simulink model "IOControls"  (R2019b)
settings: configuration reference "ConfigSet_IOControls_Reference" (kept outside this file)
model workspace (MAT data in the model file):
  SampleTime = 0.05
libraries: IOStateMachinesLib x274, SignalGeneratorsLib x1, simulink x1
(part 2 of 10)

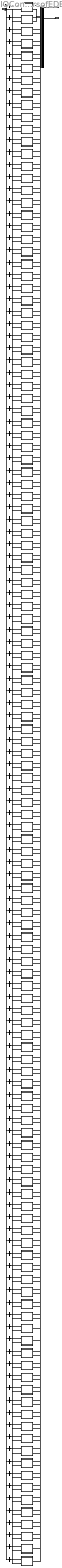
== system IOControls/ForEachVehicle/IOControls/Non-CabControl/CircuitBreakersofEDB ==
  ModelInputs : Inport
  Initialise : Inport  Port=2
  AC1CB : Subsystem  mask{InitState=1, ControlStates=[0,1], OnStateValue=1, OffStateValue=0}
      mask prompts: InitState "Initial State"; ControlStates "Software State Values"; OnStateValue "On State Value"; OffStateValue "Off State Value"
  AC2CB : Subsystem  mask{InitState=1, ControlStates=[0,1], OnStateValue=1, OffStateValue=0}
      mask prompts: InitState "Initial State"; ControlStates "Software State Values"; OnStateValue "On State Value"; OffStateValue "Off State Value"
  ADDCOS : Subsystem  mask{InitState=0, ControlStates=[0,1], OnStateValue=1, OffStateValue=0}
      mask prompts: InitState "Initial State"; ControlStates "Software State Values"; OnStateValue "On State Value"; OffStateValue "Off State Value"
  APSCB : Subsystem  mask{InitState=1, ControlStates=[0,1], OnStateValue=1, OffStateValue=0}
      mask prompts: InitState "Initial State"; ControlStates "Software State Values"; OnStateValue "On State Value"; OffStateValue "Off State Value"
  APSICB : Subsystem  mask{InitState=1, ControlStates=[0,1], OnStateValue=1, OffStateValue=0}
      mask prompts: InitState "Initial State"; ControlStates "Software State Values"; OnStateValue "On State Value"; OffStateValue "Off State Value"
  BCBCB : Subsystem  mask{InitState=1, ControlStates=[0,1], OnStateValue=1, OffStateValue=0}
      mask prompts: InitState "Initial State"; ControlStates "Software State Values"; OnStateValue "On State Value"; OffStateValue "Off State Value"
  BCGCB : Subsystem  mask{InitState=1, ControlStates=[0,1], OnStateValue=1, OffStateValue=0}
      mask prompts: InitState "Initial State"; ControlStates "Software State Values"; OnStateValue "On State Value"; OffStateValue "Off State Value"
  BC_Inputs : BusCreator  Inputs=128
  BC_MCBTrip : BusCreator  Inputs=124
  BECUCB1 : Subsystem  mask{InitState=1, ControlStates=[0,1], OnStateValue=1, OffStateValue=0}
      mask prompts: InitState "Initial State"; ControlStates "Software State Values"; OnStateValue "On State Value"; OffStateValue "Off State Value"
  BECUCB2 : Subsystem  mask{InitState=1, ControlStates=[0,1], OnStateValue=1, OffStateValue=0}
      mask prompts: InitState "Initial State"; ControlStates "Software State Values"; OnStateValue "On State Value"; OffStateValue "Off State Value"
  BECUCB3 : Subsystem  mask{InitState=1, ControlStates=[0,1], OnStateValue=1, OffStateValue=0}
      mask prompts: InitState "Initial State"; ControlStates "Software State Values"; OnStateValue "On State Value"; OffStateValue "Off State Value"
  BLCB : Subsystem  mask{InitState=1, ControlStates=[0,1], OnStateValue=1, OffStateValue=0}
      mask prompts: InitState "Initial State"; ControlStates "Software State Values"; OnStateValue "On State Value"; OffStateValue "Off State Value"
  BS_Control1 : BusSelector  OutputSignals=EBLR2CB
  BS_Control10 : BusSelector  OutputSignals=ILCB1
  BS_Control100 : BusSelector  OutputSignals=SP3CB
  BS_Control101 : BusSelector  OutputSignals=SP4CB
  BS_Control102 : BusSelector  OutputSignals=SP5CB
  BS_Control103 : BusSelector  OutputSignals=SPCB6
  BS_Control104 : BusSelector  OutputSignals=SPCB7
  BS_Control105 : BusSelector  OutputSignals=SPCB8
  BS_Control106 : BusSelector  OutputSignals=RPTCB
  BS_Control107 : BusSelector  OutputSignals=TERCB1
  BS_Control108 : BusSelector  OutputSignals=TERCB2
  BS_Control109 : BusSelector  OutputSignals=SPSW
  BS_Control11 : BusSelector  OutputSignals=ILCB2
  BS_Control110 : BusSelector  OutputSignals=SPPB
  BS_Control111 : BusSelector  OutputSignals=APSCB
  BS_Control112 : BusSelector  OutputSignals=APSICB
  BS_Control113 : BusSelector  OutputSignals=BCGCB
  BS_Control114 : BusSelector  OutputSignals=DSCB
  BS_Control115 : BusSelector  OutputSignals=MTBMCCB
  BS_Control116 : BusSelector  OutputSignals=PADCB
  BS_Control117 : BusSelector  OutputSignals=PANCB
  BS_Control118 : BusSelector  OutputSignals=SSCB
  BS_Control119 : BusSelector  OutputSignals=PTCB
  BS_Control12 : BusSelector  OutputSignals=LDICB
  BS_Control120 : BusSelector  OutputSignals=VCBCB
  BS_Control121 : BusSelector  OutputSignals=SP12CB
  BS_Control122 : BusSelector  OutputSignals=MTBM1CB
  BS_Control123 : BusSelector  OutputSignals=MTBM2CB
  BS_Control124 : BusSelector  OutputSignals=SP11CB
  BS_Control125 : BusSelector  OutputSignals=SP6CB
  BS_Control126 : BusSelector  OutputSignals=MTOPCB
  BS_Control127 : BusSelector  OutputSignals=ORDCOS
  BS_Control128 : BusSelector  OutputSignals=ADDCOS
  BS_Control13 : BusSelector  OutputSignals=LDLCB
  BS_Control14 : BusSelector  OutputSignals=LDRCB
  BS_Control15 : BusSelector  OutputSignals=MLCB
  BS_Control16 : BusSelector  OutputSignals=MMCB
  BS_Control17 : BusSelector  OutputSignals=NBCB
  BS_Control18 : BusSelector  OutputSignals=NVICB
  BS_Control19 : BusSelector  OutputSignals=OCCB1
  BS_Control2 : BusSelector  OutputSignals=EBMVCB
  BS_Control20 : BusSelector  OutputSignals=OCCB2
  BS_Control21 : BusSelector  OutputSignals=ODDCB
  BS_Control22 : BusSelector  OutputSignals=PBCB
  BS_Control23 : BusSelector  OutputSignals=PISCB1
  BS_Control24 : BusSelector  OutputSignals=PISCB2
  BS_Control25 : BusSelector  OutputSignals=POCB
  BS_Control26 : BusSelector  OutputSignals=PPU1CB
  BS_Control27 : BusSelector  OutputSignals=PPU2CB
  BS_Control28 : BusSelector  OutputSignals=PPU3CB
  BS_Control29 : BusSelector  OutputSignals=RIO1CB
  BS_Control3 : BusSelector  OutputSignals=EDCB
  BS_Control30 : BusSelector  OutputSignals=RIO2CB
  BS_Control31 : BusSelector  OutputSignals=SIOCB1
  BS_Control32 : BusSelector  OutputSignals=SIOCB2
  BS_Control33 : BusSelector  OutputSignals=SSICB
  BS_Control34 : BusSelector  OutputSignals=TBCCB1
  BS_Control35 : BusSelector  OutputSignals=TBCCB2
  BS_Control36 : BusSelector  OutputSignals=TBNCB
  BS_Control37 : BusSelector  OutputSignals=TDICB
  BS_Control38 : BusSelector  OutputSignals=TLLCB
  BS_Control39 : BusSelector  OutputSignals=TLRCB
  BS_Control4 : BusSelector  OutputSignals=ELCB1
  BS_Control40 : BusSelector  OutputSignals=TRIVCB
  BS_Control41 : BusSelector  OutputSignals=TVDUCB
  BS_Control42 : BusSelector  OutputSignals=TWVCB
  BS_Control43 : BusSelector  OutputSignals=VCCBOrUCCB
  BS_Control44 : BusSelector  OutputSignals=VCBCCB
  BS_Control45 : BusSelector  OutputSignals=VIO1CB
  BS_Control46 : BusSelector  OutputSignals=VIO2CB
  BS_Control47 : BusSelector  OutputSignals=WFLCB
  BS_Control48 : BusSelector  OutputSignals=WIFICB
  BS_Control49 : BusSelector  OutputSignals=WWCB
  BS_Control5 : BusSelector  OutputSignals=ELCB2
  BS_Control50 : BusSelector  OutputSignals=BECUCB1
  BS_Control51 : BusSelector  OutputSignals=BECUCB2
  BS_Control52 : BusSelector  OutputSignals=BECUCB3
  BS_Control53 : BusSelector  OutputSignals=RSACB
  BS_Control54 : BusSelector  OutputSignals=CMCCB
  BS_Control55 : BusSelector  OutputSignals=CILCB
  BS_Control56 : BusSelector  OutputSignals=CICB
  BS_Control57 : BusSelector  OutputSignals=CELCB
  BS_Control58 : BusSelector  OutputSignals=CECB
  BS_Control59 : BusSelector  OutputSignals=CDUCB
  BS_Control6 : BusSelector  OutputSignals=ERCB
  BS_Control60 : BusSelector  OutputSignals=CCNVIO1CB
  BS_Control61 : BusSelector  OutputSignals=CBTCCB1
  BS_Control62 : BusSelector  OutputSignals=CBFCCB
  BS_Control63 : BusSelector  OutputSignals=CBFCB
  BS_Control64 : BusSelector  OutputSignals=C1CB
  BS_Control65 : BusSelector  OutputSignals=BLCB
  BS_Control66 : BusSelector  OutputSignals=ZVBACB
  BS_Control67 : BusSelector  OutputSignals=EBLR1CB
  BS_Control68 : BusSelector  OutputSignals=DRCB
  BS_Control69 : BusSelector  OutputSignals=DPLCB
  BS_Control7 : BusSelector  OutputSignals=HCB
  BS_Control70 : BusSelector  OutputSignals=DMICB
  BS_Control71 : BusSelector  OutputSignals=DLCB
  BS_Control72 : BusSelector  OutputSignals=DIOCB2
  BS_Control73 : BusSelector  OutputSignals=DIOCB1
  BS_Control74 : BusSelector  OutputSignals=CSCCB
  BS_Control75 : BusSelector  OutputSignals=CSBCB
  BS_Control76 : BusSelector  OutputSignals=CSACB
  BS_Control77 : BusSelector  OutputSignals=CRSBCB
  BS_Control78 : BusSelector  OutputSignals=SOCB2
  BS_Control79 : BusSelector  OutputSignals=SOCB1
  BS_Control8 : BusSelector  OutputSignals=HLLCB
  BS_Control80 : BusSelector  OutputSignals=MSOCB5
  BS_Control81 : BusSelector  OutputSignals=MSOCB4
  BS_Control82 : BusSelector  OutputSignals=MSOCB3
  BS_Control83 : BusSelector  OutputSignals=MSOCB2
  BS_Control84 : BusSelector  OutputSignals=MSOCB1
  BS_Control85 : BusSelector  OutputSignals=HVAC1
  BS_Control86 : BusSelector  OutputSignals=SAC2CCB
  BS_Control87 : BusSelector  OutputSignals=HVAC2
  BS_Control88 : BusSelector  OutputSignals=SAC1CCB
  BS_Control89 : BusSelector  OutputSignals=CMCB
  BS_Control9 : BusSelector  OutputSignals=HLRCB
  BS_Control90 : BusSelector  OutputSignals=AC2CB
  BS_Control91 : BusSelector  OutputSignals=AC1CB
  BS_Control92 : BusSelector  OutputSignals=FDSCB
  BS_Control93 : BusSelector  OutputSignals=BCBCB
  BS_Control94 : BusSelector  OutputSignals=ERVRCB1
  BS_Control95 : BusSelector  OutputSignals=ERVRCB2
  BS_Control96 : BusSelector  OutputSignals=ESKCB
  BS_Control97 : BusSelector  OutputSignals=HMCB
  BS_Control98 : BusSelector  OutputSignals=SP1CB
  BS_Control99 : BusSelector  OutputSignals=SP2CB
  C1CB : Subsystem  mask{InitState=1, ControlStates=[0,1], OnStateValue=1, OffStateValue=0}
      mask prompts: InitState "Initial State"; ControlStates "Software State Values"; OnStateValue "On State Value"; OffStateValue "Off State Value"
  CBFCB : Subsystem  mask{InitState=1, ControlStates=[0,1], OnStateValue=1, OffStateValue=0}
      mask prompts: InitState "Initial State"; ControlStates "Software State Values"; OnStateValue "On State Value"; OffStateValue "Off State Value"
  CBFCCB : Subsystem  mask{InitState=1, ControlStates=[0,1], OnStateValue=1, OffStateValue=0}
      mask prompts: InitState "Initial State"; ControlStates "Software State Values"; OnStateValue "On State Value"; OffStateValue "Off State Value"
  CBTCCB1 : Subsystem  mask{InitState=1, ControlStates=[0,1], OnStateValue=1, OffStateValue=0}
      mask prompts: InitState "Initial State"; ControlStates "Software State Values"; OnStateValue "On State Value"; OffStateValue "Off State Value"
  CCNVIO1CB : Subsystem  mask{InitState=1, ControlStates=[0,1], OnStateValue=1, OffStateValue=0}
      mask prompts: InitState "Initial State"; ControlStates "Software State Values"; OnStateValue "On State Value"; OffStateValue "Off State Value"
  CDUCB : Subsystem  mask{InitState=1, ControlStates=[0,1], OnStateValue=1, OffStateValue=0}
      mask prompts: InitState "Initial State"; ControlStates "Software State Values"; OnStateValue "On State Value"; OffStateValue "Off State Value"
  CECB : Subsystem  mask{InitState=1, ControlStates=[0,1], OnStateValue=1, OffStateValue=0}
      mask prompts: InitState "Initial State"; ControlStates "Software State Values"; OnStateValue "On State Value"; OffStateValue "Off State Value"
  CELCB : Subsystem  mask{InitState=1, ControlStates=[0,1], OnStateValue=1, OffStateValue=0}
      mask prompts: InitState "Initial State"; ControlStates "Software State Values"; OnStateValue "On State Value"; OffStateValue "Off State Value"
  CICB : Subsystem  mask{InitState=1, ControlStates=[0,1], OnStateValue=1, OffStateValue=0}
      mask prompts: InitState "Initial State"; ControlStates "Software State Values"; OnStateValue "On State Value"; OffStateValue "Off State Value"
  CILCB : Subsystem  mask{InitState=1, ControlStates=[0,1], OnStateValue=1, OffStateValue=0}
      mask prompts: InitState "Initial State"; ControlStates "Software State Values"; OnStateValue "On State Value"; OffStateValue "Off State Value"
  CMCB : Subsystem  mask{InitState=1, ControlStates=[0,1], OnStateValue=1, OffStateValue=0}
      mask prompts: InitState "Initial State"; ControlStates "Software State Values"; OnStateValue "On State Value"; OffStateValue "Off State Value"
  CMCCB : Subsystem  mask{InitState=1, ControlStates=[0,1], OnStateValue=1, OffStateValue=0}
      mask prompts: InitState "Initial State"; ControlStates "Software State Values"; OnStateValue "On State Value"; OffStateValue "Off State Value"
  CRSBCB : Subsystem  mask{InitState=1, ControlStates=[0,1], OnStateValue=1, OffStateValue=0}
      mask prompts: InitState "Initial State"; ControlStates "Software State Values"; OnStateValue "On State Value"; OffStateValue "Off State Value"
  CSACB : Subsystem  mask{InitState=1, ControlStates=[0,1], OnStateValue=1, OffStateValue=0}
      mask prompts: InitState "Initial State"; ControlStates "Software State Values"; OnStateValue "On State Value"; OffStateValue "Off State Value"
  CSBCB : Subsystem  mask{InitState=1, ControlStates=[0,1], OnStateValue=1, OffStateValue=0}
      mask prompts: InitState "Initial State"; ControlStates "Software State Values"; OnStateValue "On State Value"; OffStateValue "Off State Value"
  CSCCB : Subsystem  mask{InitState=1, ControlStates=[0,1], OnStateValue=1, OffStateValue=0}
      mask prompts: InitState "Initial State"; ControlStates "Software State Values"; OnStateValue "On State Value"; OffStateValue "Off State Value"
  DIOCB1 : Subsystem  mask{InitState=1, ControlStates=[0,1], OnStateValue=1, OffStateValue=0}
      mask prompts: InitState "Initial State"; ControlStates "Software State Values"; OnStateValue "On State Value"; OffStateValue "Off State Value"
  DIOCB2 : Subsystem  mask{InitState=1, ControlStates=[0,1], OnStateValue=1, OffStateValue=0}
      mask prompts: InitState "Initial State"; ControlStates "Software State Values"; OnStateValue "On State Value"; OffStateValue "Off State Value"
  DLCB : Subsystem  mask{InitState=1, ControlStates=[0,1], OnStateValue=1, OffStateValue=0}
      mask prompts: InitState "Initial State"; ControlStates "Software State Values"; OnStateValue "On State Value"; OffStateValue "Off State Value"
  DMICB : Subsystem  mask{InitState=1, ControlStates=[0,1], OnStateValue=1, OffStateValue=0}
      mask prompts: InitState "Initial State"; ControlStates "Software State Values"; OnStateValue "On State Value"; OffStateValue "Off State Value"
  DPLCB : Subsystem  mask{InitState=1, ControlStates=[0,1], OnStateValue=1, OffStateValue=0}
      mask prompts: InitState "Initial State"; ControlStates "Software State Values"; OnStateValue "On State Value"; OffStateValue "Off State Value"
  DRCB : Subsystem  mask{InitState=1, ControlStates=[0,1], OnStateValue=1, OffStateValue=0}
      mask prompts: InitState "Initial State"; ControlStates "Software State Values"; OnStateValue "On State Value"; OffStateValue "Off State Value"
  DSCB : Subsystem  mask{InitState=1, ControlStates=[0,1], OnStateValue=1, OffStateValue=0}
      mask prompts: InitState "Initial State"; ControlStates "Software State Values"; OnStateValue "On State Value"; OffStateValue "Off State Value"
  EBLR1CB : Subsystem  mask{InitState=1, ControlStates=[0,1], OnStateValue=1, OffStateValue=0}
      mask prompts: InitState "Initial State"; ControlStates "Software State Values"; OnStateValue "On State Value"; OffStateValue "Off State Value"
  EBLR2CB : Subsystem  mask{InitState=1, ControlStates=[0,1], OnStateValue=1, OffStateValue=0}
      mask prompts: InitState "Initial State"; ControlStates "Software State Values"; OnStateValue "On State Value"; OffStateValue "Off State Value"
  EBMVCB : Subsystem  mask{InitState=1, ControlStates=[0,1], OnStateValue=1, OffStateValue=0}
      mask prompts: InitState "Initial State"; ControlStates "Software State Values"; OnStateValue "On State Value"; OffStateValue "Off State Value"
  EDCB : Subsystem  mask{InitState=1, ControlStates=[0,1], OnStateValue=1, OffStateValue=0}
      mask prompts: InitState "Initial State"; ControlStates "Software State Values"; OnStateValue "On State Value"; OffStateValue "Off State Value"
  ELCB1 : Subsystem  mask{InitState=1, ControlStates=[0,1], OnStateValue=1, OffStateValue=0}
      mask prompts: InitState "Initial State"; ControlStates "Software State Values"; OnStateValue "On State Value"; OffStateValue "Off State Value"
  ELCB2 : Subsystem  mask{InitState=1, ControlStates=[0,1], OnStateValue=1, OffStateValue=0}
      mask prompts: InitState "Initial State"; ControlStates "Software State Values"; OnStateValue "On State Value"; OffStateValue "Off State Value"
  ERCB : Subsystem  mask{InitState=1, ControlStates=[0,1], OnStateValue=1, OffStateValue=0}
      mask prompts: InitState "Initial State"; ControlStates "Software State Values"; OnStateValue "On State Value"; OffStateValue "Off State Value"
  ERVRCB1 : Subsystem  mask{InitState=1, ControlStates=[0,1], OnStateValue=1, OffStateValue=0}
      mask prompts: InitState "Initial State"; ControlStates "Software State Values"; OnStateValue "On State Value"; OffStateValue "Off State Value"
  ERVRCB2 : Subsystem  mask{InitState=1, ControlStates=[0,1], OnStateValue=1, OffStateValue=0}
      mask prompts: InitState "Initial State"; ControlStates "Software State Values"; OnStateValue "On State Value"; OffStateValue "Off State Value"
  ESKCB : Subsystem  mask{InitState=1, ControlStates=[0,1], OnStateValue=1, OffStateValue=0}
      mask prompts: InitState "Initial State"; ControlStates "Software State Values"; OnStateValue "On State Value"; OffStateValue "Off State Value"
  FDSCB : Subsystem  mask{InitState=1, ControlStates=[0,1], OnStateValue=1, OffStateValue=0}
      mask prompts: InitState "Initial State"; ControlStates "Software State Values"; OnStateValue "On State Value"; OffStateValue "Off State Value"
  HCB : Subsystem  mask{InitState=1, ControlStates=[0,1], OnStateValue=1, OffStateValue=0}
      mask prompts: InitState "Initial State"; ControlStates "Software State Values"; OnStateValue "On State Value"; OffStateValue "Off State Value"
  HLLCB : Subsystem  mask{InitState=1, ControlStates=[0,1], OnStateValue=1, OffStateValue=0}
      mask prompts: InitState "Initial State"; ControlStates "Software State Values"; OnStateValue "On State Value"; OffStateValue "Off State Value"
  HLRCB : Subsystem  mask{InitState=1, ControlStates=[0,1], OnStateValue=1, OffStateValue=0}
      mask prompts: InitState "Initial State"; ControlStates "Software State Values"; OnStateValue "On State Value"; OffStateValue "Off State Value"
  HMCB : Subsystem  mask{InitState=1, ControlStates=[0,1], OnStateValue=1, OffStateValue=0}
      mask prompts: InitState "Initial State"; ControlStates "Software State Values"; OnStateValue "On State Value"; OffStateValue "Off State Value"
  HVAC1 : Subsystem  mask{InitState=1, ControlStates=[0,1], OnStateValue=1, OffStateValue=0}
      mask prompts: InitState "Initial State"; ControlStates "Software State Values"; OnStateValue "On State Value"; OffStateValue "Off State Value"
  HVAC2 : Subsystem  mask{InitState=1, ControlStates=[0,1], OnStateValue=1, OffStateValue=0}
      mask prompts: InitState "Initial State"; ControlStates "Software State Values"; OnStateValue "On State Value"; OffStateValue "Off State Value"
  ILCB1 : Subsystem  mask{InitState=1, ControlStates=[0,1], OnStateValue=1, OffStateValue=0}
      mask prompts: InitState "Initial State"; ControlStates "Software State Values"; OnStateValue "On State Value"; OffStateValue "Off State Value"
  ILCB2 : Subsystem  mask{InitState=1, ControlStates=[0,1], OnStateValue=1, OffStateValue=0}
      mask prompts: InitState "Initial State"; ControlStates "Software State Values"; OnStateValue "On State Value"; OffStateValue "Off State Value"
  LDICB : Subsystem  mask{InitState=1, ControlStates=[0,1], OnStateValue=1, OffStateValue=0}
      mask prompts: InitState "Initial State"; ControlStates "Software State Values"; OnStateValue "On State Value"; OffStateValue "Off State Value"
  LDLCB : Subsystem  mask{InitState=1, ControlStates=[0,1], OnStateValue=1, OffStateValue=0}
      mask prompts: InitState "Initial State"; ControlStates "Software State Values"; OnStateValue "On State Value"; OffStateValue "Off State Value"
  LDRCB : Subsystem  mask{InitState=1, ControlStates=[0,1], OnStateValue=1, OffStateValue=0}
      mask prompts: InitState "Initial State"; ControlStates "Software State Values"; OnStateValue "On State Value"; OffStateValue "Off State Value"
  MLCB : Subsystem  mask{InitState=1, ControlStates=[0,1], OnStateValue=1, OffStateValue=0}
      mask prompts: InitState "Initial State"; ControlStates "Software State Values"; OnStateValue "On State Value"; OffStateValue "Off State Value"
  MMCB : Subsystem  mask{InitState=1, ControlStates=[0,1], OnStateValue=1, OffStateValue=0}
      mask prompts: InitState "Initial State"; ControlStates "Software State Values"; OnStateValue "On State Value"; OffStateValue "Off State Value"
  MSOCB1 : Subsystem  mask{InitState=1, ControlStates=[0,1], OnStateValue=1, OffStateValue=0}
      mask prompts: InitState "Initial State"; ControlStates "Software State Values"; OnStateValue "On State Value"; OffStateValue "Off State Value"
  MSOCB2 : Subsystem  mask{InitState=1, ControlStates=[0,1], OnStateValue=1, OffStateValue=0}
      mask prompts: InitState "Initial State"; ControlStates "Software State Values"; OnStateValue "On State Value"; OffStateValue "Off State Value"
  MSOCB3 : Subsystem  mask{InitState=1, ControlStates=[0,1], OnStateValue=1, OffStateValue=0}
      mask prompts: InitState "Initial State"; ControlStates "Software State Values"; OnStateValue "On State Value"; OffStateValue "Off State Value"
  MSOCB4 : Subsystem  mask{InitState=1, ControlStates=[0,1], OnStateValue=1, OffStateValue=0}
      mask prompts: InitState "Initial State"; ControlStates "Software State Values"; OnStateValue "On State Value"; OffStateValue "Off State Value"
  MSOCB5 : Subsystem  mask{InitState=1, ControlStates=[0,1], OnStateValue=1, OffStateValue=0}
      mask prompts: InitState "Initial State"; ControlStates "Software State Values"; OnStateValue "On State Value"; OffStateValue "Off State Value"
  MTBM1CB : Subsystem  mask{InitState=1, ControlStates=[0,1], OnStateValue=1, OffStateValue=0}
      mask prompts: InitState "Initial State"; ControlStates "Software State Values"; OnStateValue "On State Value"; OffStateValue "Off State Value"
  MTBM2CB : Subsystem  mask{InitState=1, ControlStates=[0,1], OnStateValue=1, OffStateValue=0}
      mask prompts: InitState "Initial State"; ControlStates "Software State Values"; OnStateValue "On State Value"; OffStateValue "Off State Value"
  MTBMCCB : Subsystem  mask{InitState=1, ControlStates=[0,1], OnStateValue=1, OffStateValue=0}
      mask prompts: InitState "Initial State"; ControlStates "Software State Values"; OnStateValue "On State Value"; OffStateValue "Off State Value"
  MTOPCB : Subsystem  mask{InitState=1, ControlStates=[0,1], OnStateValue=1, OffStateValue=0}
      mask prompts: InitState "Initial State"; ControlStates "Software State Values"; OnStateValue "On State Value"; OffStateValue "Off State Value"
  NBCB : Subsystem  mask{InitState=1, ControlStates=[0,1], OnStateValue=1, OffStateValue=0}
      mask prompts: InitState "Initial State"; ControlStates "Software State Values"; OnStateValue "On State Value"; OffStateValue "Off State Value"
  NVICB : Subsystem  mask{InitState=1, ControlStates=[0,1], OnStateValue=1, OffStateValue=0}
      mask prompts: InitState "Initial State"; ControlStates "Software State Values"; OnStateValue "On State Value"; OffStateValue "Off State Value"
  OCCB1 : Subsystem  mask{InitState=1, ControlStates=[0,1], OnStateValue=1, OffStateValue=0}
      mask prompts: InitState "Initial State"; ControlStates "Software State Values"; OnStateValue "On State Value"; OffStateValue "Off State Value"
  OCCB2 : Subsystem  mask{InitState=1, ControlStates=[0,1], OnStateValue=1, OffStateValue=0}
      mask prompts: InitState "Initial State"; ControlStates "Software State Values"; OnStateValue "On State Value"; OffStateValue "Off State Value"
  ODDCB : Subsystem  mask{InitState=1, ControlStates=[0,1], OnStateValue=1, OffStateValue=0}
      mask prompts: InitState "Initial State"; ControlStates "Software State Values"; OnStateValue "On State Value"; OffStateValue "Off State Value"
  ORDCOS : Subsystem  mask{InitState=0, ControlStates=[0,1], OnStateValue=1, OffStateValue=0}
      mask prompts: InitState "Initial State"; ControlStates "Software State Values"; OnStateValue "On State Value"; OffStateValue "Off State Value"
  PADCB : Subsystem  mask{InitState=1, ControlStates=[0,1], OnStateValue=1, OffStateValue=0}
      mask prompts: InitState "Initial State"; ControlStates "Software State Values"; OnStateValue "On State Value"; OffStateValue "Off State Value"
  PANCB : Subsystem  mask{InitState=1, ControlStates=[0,1], OnStateValue=1, OffStateValue=0}
      mask prompts: InitState "Initial State"; ControlStates "Software State Values"; OnStateValue "On State Value"; OffStateValue "Off State Value"
  PBCB : Subsystem  mask{InitState=1, ControlStates=[0,1], OnStateValue=1, OffStateValue=0}
      mask prompts: InitState "Initial State"; ControlStates "Software State Values"; OnStateValue "On State Value"; OffStateValue "Off State Value"
  PISCB1 : Subsystem  mask{InitState=1, ControlStates=[0,1], OnStateValue=1, OffStateValue=0}
      mask prompts: InitState "Initial State"; ControlStates "Software State Values"; OnStateValue "On State Value"; OffStateValue "Off State Value"
  PISCB2 : Subsystem  mask{InitState=1, ControlStates=[0,1], OnStateValue=1, OffStateValue=0}
      mask prompts: InitState "Initial State"; ControlStates "Software State Values"; OnStateValue "On State Value"; OffStateValue "Off State Value"
  POCB : Subsystem  mask{InitState=1, ControlStates=[0,1], OnStateValue=1, OffStateValue=0}
      mask prompts: InitState "Initial State"; ControlStates "Software State Values"; OnStateValue "On State Value"; OffStateValue "Off State Value"
  PPU1CB : Subsystem  mask{InitState=1, ControlStates=[0,1], OnStateValue=1, OffStateValue=0}
      mask prompts: InitState "Initial State"; ControlStates "Software State Values"; OnStateValue "On State Value"; OffStateValue "Off State Value"
  PPU2CB : Subsystem  mask{InitState=1, ControlStates=[0,1], OnStateValue=1, OffStateValue=0}
      mask prompts: InitState "Initial State"; ControlStates "Software State Values"; OnStateValue "On State Value"; OffStateValue "Off State Value"
  PPU3CB : Subsystem  mask{InitState=1, ControlStates=[0,1], OnStateValue=1, OffStateValue=0}
      mask prompts: InitState "Initial State"; ControlStates "Software State Values"; OnStateValue "On State Value"; OffStateValue "Off State Value"
  PTCB : Subsystem  mask{InitState=1, ControlStates=[0,1], OnStateValue=1, OffStateValue=0}
      mask prompts: InitState "Initial State"; ControlStates "Software State Values"; OnStateValue "On State Value"; OffStateValue "Off State Value"
  RIO1CB : Subsystem  mask{InitState=1, ControlStates=[0,1], OnStateValue=1, OffStateValue=0}
      mask prompts: InitState "Initial State"; ControlStates "Software State Values"; OnStateValue "On State Value"; OffStateValue "Off State Value"
  RIO2CB : Subsystem  mask{InitState=1, ControlStates=[0,1], OnStateValue=1, OffStateValue=0}
      mask prompts: InitState "Initial State"; ControlStates "Software State Values"; OnStateValue "On State Value"; OffStateValue "Off State Value"
  RPTCB : Subsystem  mask{InitState=1, ControlStates=[0,1], OnStateValue=1, OffStateValue=0}
      mask prompts: InitState "Initial State"; ControlStates "Software State Values"; OnStateValue "On State Value"; OffStateValue "Off State Value"
  RSACB : Subsystem  mask{InitState=1, ControlStates=[0,1], OnStateValue=1, OffStateValue=0}
      mask prompts: InitState "Initial State"; ControlStates "Software State Values"; OnStateValue "On State Value"; OffStateValue "Off State Value"
  SAC1CCB : Subsystem  mask{InitState=1, ControlStates=[0,1], OnStateValue=1, OffStateValue=0}
      mask prompts: InitState "Initial State"; ControlStates "Software State Values"; OnStateValue "On State Value"; OffStateValue "Off State Value"
  SAC2CCB : Subsystem  mask{InitState=1, ControlStates=[0,1], OnStateValue=1, OffStateValue=0}
      mask prompts: InitState "Initial State"; ControlStates "Software State Values"; OnStateValue "On State Value"; OffStateValue "Off State Value"
  SIOCB1 : Subsystem  mask{InitState=1, ControlStates=[0,1], OnStateValue=1, OffStateValue=0}
      mask prompts: InitState "Initial State"; ControlStates "Software State Values"; OnStateValue "On State Value"; OffStateValue "Off State Value"
  SIOCB2 : Subsystem  mask{InitState=1, ControlStates=[0,1], OnStateValue=1, OffStateValue=0}
      mask prompts: InitState "Initial State"; ControlStates "Software State Values"; OnStateValue "On State Value"; OffStateValue "Off State Value"
  SOCB1 : Subsystem  mask{InitState=1, ControlStates=[0,1], OnStateValue=1, OffStateValue=0}
      mask prompts: InitState "Initial State"; ControlStates "Software State Values"; OnStateValue "On State Value"; OffStateValue "Off State Value"
  SOCB2 : Subsystem  mask{InitState=1, ControlStates=[0,1], OnStateValue=1, OffStateValue=0}
      mask prompts: InitState "Initial State"; ControlStates "Software State Values"; OnStateValue "On State Value"; OffStateValue "Off State Value"
  SP11CB : Subsystem  mask{InitState=1, ControlStates=[0,1], OnStateValue=1, OffStateValue=0}
      mask prompts: InitState "Initial State"; ControlStates "Software State Values"; OnStateValue "On State Value"; OffStateValue "Off State Value"
  SP12CB : Subsystem  mask{InitState=1, ControlStates=[0,1], OnStateValue=1, OffStateValue=0}
      mask prompts: InitState "Initial State"; ControlStates "Software State Values"; OnStateValue "On State Value"; OffStateValue "Off State Value"
  SP1CB : Subsystem  mask{InitState=1, ControlStates=[0,1], OnStateValue=1, OffStateValue=0}
      mask prompts: InitState "Initial State"; ControlStates "Software State Values"; OnStateValue "On State Value"; OffStateValue "Off State Value"
  SP2CB : Subsystem  mask{InitState=1, ControlStates=[0,1], OnStateValue=1, OffStateValue=0}
      mask prompts: InitState "Initial State"; ControlStates "Software State Values"; OnStateValue "On State Value"; OffStateValue "Off State Value"
  SP3CB : Subsystem  mask{InitState=1, ControlStates=[0,1], OnStateValue=1, OffStateValue=0}
      mask prompts: InitState "Initial State"; ControlStates "Software State Values"; OnStateValue "On State Value"; OffStateValue "Off State Value"
  SP4CB : Subsystem  mask{InitState=1, ControlStates=[0,1], OnStateValue=1, OffStateValue=0}
      mask prompts: InitState "Initial State"; ControlStates "Software State Values"; OnStateValue "On State Value"; OffStateValue "Off State Value"
  SP5CB : Subsystem  mask{InitState=1, ControlStates=[0,1], OnStateValue=1, OffStateValue=0}
      mask prompts: InitState "Initial State"; ControlStates "Software State Values"; OnStateValue "On State Value"; OffStateValue "Off State Value"
  SP6CB : Subsystem  mask{InitState=1, ControlStates=[0,1], OnStateValue=1, OffStateValue=0}
      mask prompts: InitState "Initial State"; ControlStates "Software State Values"; OnStateValue "On State Value"; OffStateValue "Off State Value"
  SPCB6 : Subsystem  mask{InitState=1, ControlStates=[0,1], OnStateValue=1, OffStateValue=0}
      mask prompts: InitState "Initial State"; ControlStates "Software State Values"; OnStateValue "On State Value"; OffStateValue "Off State Value"
  SPCB7 : Subsystem  mask{InitState=1, ControlStates=[0,1], OnStateValue=1, OffStateValue=0}
      mask prompts: InitState "Initial State"; ControlStates "Software State Values"; OnStateValue "On State Value"; OffStateValue "Off State Value"
  SPCB8 : Subsystem  mask{InitState=1, ControlStates=[0,1], OnStateValue=1, OffStateValue=0}
      mask prompts: InitState "Initial State"; ControlStates "Software State Values"; OnStateValue "On State Value"; OffStateValue "Off State Value"
  SPPB : Subsystem  mask{InitState=0, ControlStates=[0,1], OnStateValue=1, OffStateValue=0}
      mask prompts: InitState "Initial State"; ControlStates "Software State Values"; OnStateValue "On State Value"; OffStateValue "Off State Value"
  SPSW : Subsystem  mask{InitState=0, ControlStates=[0,1], OnStateValue=1, OffStateValue=0}
      mask prompts: InitState "Initial State"; ControlStates "Software State Values"; OnStateValue "On State Value"; OffStateValue "Off State Value"
  SSCB : Subsystem  mask{InitState=1, ControlStates=[0,1], OnStateValue=1, OffStateValue=0}
      mask prompts: InitState "Initial State"; ControlStates "Software State Values"; OnStateValue "On State Value"; OffStateValue "Off State Value"
  SSICB : Subsystem  mask{InitState=1, ControlStates=[0,1], OnStateValue=1, OffStateValue=0}
      mask prompts: InitState "Initial State"; ControlStates "Software State Values"; OnStateValue "On State Value"; OffStateValue "Off State Value"
  TBCCB1 : Subsystem  mask{InitState=1, ControlStates=[0,1], OnStateValue=1, OffStateValue=0}
      mask prompts: InitState "Initial State"; ControlStates "Software State Values"; OnStateValue "On State Value"; OffStateValue "Off State Value"
  TBCCB2 : Subsystem  mask{InitState=1, ControlStates=[0,1], OnStateValue=1, OffStateValue=0}
      mask prompts: InitState "Initial State"; ControlStates "Software State Values"; OnStateValue "On State Value"; OffStateValue "Off State Value"
  TBNCB : Subsystem  mask{InitState=1, ControlStates=[0,1], OnStateValue=1, OffStateValue=0}
      mask prompts: InitState "Initial State"; ControlStates "Software State Values"; OnStateValue "On State Value"; OffStateValue "Off State Value"
  TDICB : Subsystem  mask{InitState=1, ControlStates=[0,1], OnStateValue=1, OffStateValue=0}
      mask prompts: InitState "Initial State"; ControlStates "Software State Values"; OnStateValue "On State Value"; OffStateValue "Off State Value"
  TERCB1 : Subsystem  mask{InitState=1, ControlStates=[0,1], OnStateValue=1, OffStateValue=0}
      mask prompts: InitState "Initial State"; ControlStates "Software State Values"; OnStateValue "On State Value"; OffStateValue "Off State Value"
  TERCB2 : Subsystem  mask{InitState=1, ControlStates=[0,1], OnStateValue=1, OffStateValue=0}
      mask prompts: InitState "Initial State"; ControlStates "Software State Values"; OnStateValue "On State Value"; OffStateValue "Off State Value"
  TLLCB : Subsystem  mask{InitState=1, ControlStates=[0,1], OnStateValue=1, OffStateValue=0}
      mask prompts: InitState "Initial State"; ControlStates "Software State Values"; OnStateValue "On State Value"; OffStateValue "Off State Value"
  TLRCB : Subsystem  mask{InitState=1, ControlStates=[0,1], OnStateValue=1, OffStateValue=0}
      mask prompts: InitState "Initial State"; ControlStates "Software State Values"; OnStateValue "On State Value"; OffStateValue "Off State Value"
  TRIVCB : Subsystem  mask{InitState=1, ControlStates=[0,1], OnStateValue=1, OffStateValue=0}
      mask prompts: InitState "Initial State"; ControlStates "Software State Values"; OnStateValue "On State Value"; OffStateValue "Off State Value"
  TVDUCB : Subsystem  mask{InitState=1, ControlStates=[0,1], OnStateValue=1, OffStateValue=0}
      mask prompts: InitState "Initial State"; ControlStates "Software State Values"; OnStateValue "On State Value"; OffStateValue "Off State Value"
  TWVCB : Subsystem  mask{InitState=1, ControlStates=[0,1], OnStateValue=1, OffStateValue=0}
      mask prompts: InitState "Initial State"; ControlStates "Software State Values"; OnStateValue "On State Value"; OffStateValue "Off State Value"
  VCBCB : Subsystem  mask{InitState=1, ControlStates=[0,1], OnStateValue=1, OffStateValue=0}
      mask prompts: InitState "Initial State"; ControlStates "Software State Values"; OnStateValue "On State Value"; OffStateValue "Off State Value"
  VCBCCB : Subsystem  mask{InitState=1, ControlStates=[0,1], OnStateValue=1, OffStateValue=0}
      mask prompts: InitState "Initial State"; ControlStates "Software State Values"; OnStateValue "On State Value"; OffStateValue "Off State Value"
  VCCBOrUCCB : Subsystem  mask{InitState=1, ControlStates=[0,1], OnStateValue=1, OffStateValue=0}
      mask prompts: InitState "Initial State"; ControlStates "Software State Values"; OnStateValue "On State Value"; OffStateValue "Off State Value"
  VIO1CB : Subsystem  mask{InitState=1, ControlStates=[0,1], OnStateValue=1, OffStateValue=0}
      mask prompts: InitState "Initial State"; ControlStates "Software State Values"; OnStateValue "On State Value"; OffStateValue "Off State Value"
  VIO2CB : Subsystem  mask{InitState=1, ControlStates=[0,1], OnStateValue=1, OffStateValue=0}
      mask prompts: InitState "Initial State"; ControlStates "Software State Values"; OnStateValue "On State Value"; OffStateValue "Off State Value"
  WFLCB : Subsystem  mask{InitState=1, ControlStates=[0,1], OnStateValue=1, OffStateValue=0}
      mask prompts: InitState "Initial State"; ControlStates "Software State Values"; OnStateValue "On State Value"; OffStateValue "Off State Value"
  WIFICB : Subsystem  mask{InitState=1, ControlStates=[0,1], OnStateValue=1, OffStateValue=0}
      mask prompts: InitState "Initial State"; ControlStates "Software State Values"; OnStateValue "On State Value"; OffStateValue "Off State Value"
  WWCB : Subsystem  mask{InitState=1, ControlStates=[0,1], OnStateValue=1, OffStateValue=0}
      mask prompts: InitState "Initial State"; ControlStates "Software State Values"; OnStateValue "On State Value"; OffStateValue "Off State Value"
  ZVBACB : Subsystem  mask{InitState=1, ControlStates=[0,1], OnStateValue=1, OffStateValue=0}
      mask prompts: InitState "Initial State"; ControlStates "Software State Values"; OnStateValue "On State Value"; OffStateValue "Off State Value"
  TierControlsInputs : Outport  VectorParamsAs1DForOutWhenUnconnected=off
  TierControlsMCBTrip : Outport  Port=2  VectorParamsAs1DForOutWhenUnconnected=off
  wires:
  BC_MCBTrip/1 -> TierControlsMCBTrip/1  "CircuitBreakersofEDB"
  BC_Inputs/1 -> TierControlsInputs/1  "CircuitBreakersofEDB"
  ModelInputs/1 -> BS_Control1/1, BS_Control2/1, BS_Control3/1, BS_Control4/1, BS_Control5/1, BS_Control6/1, BS_Control7/1, BS_Control8/1, BS_Control9/1, BS_Control10/1, BS_Control11/1, BS_Control12/1, BS_Control13/1, BS_Control14/1, BS_Control15/1, BS_Control16/1, BS_Control17/1, BS_Control18/1, BS_Control19/1, BS_Control20/1, BS_Control21/1, BS_Control22/1, BS_Control23/1, BS_Control24/1, BS_Control25/1, BS_Control26/1, BS_Control27/1, BS_Control28/1, BS_Control29/1, BS_Control30/1, BS_Control31/1, BS_Control32/1, BS_Control33/1, BS_Control34/1, BS_Control35/1, BS_Control36/1, BS_Control37/1, BS_Control38/1, BS_Control39/1, BS_Control40/1, BS_Control41/1, BS_Control42/1, BS_Control43/1, BS_Control44/1, BS_Control45/1, BS_Control46/1, BS_Control47/1, BS_Control48/1, BS_Control49/1, BS_Control50/1, BS_Control51/1, BS_Control52/1, BS_Control53/1, BS_Control54/1, BS_Control55/1, BS_Control56/1, BS_Control57/1, BS_Control58/1, BS_Control59/1, BS_Control60/1, BS_Control61/1, BS_Control62/1, BS_Control63/1, BS_Control64/1, BS_Control65/1, BS_Control66/1, BS_Control67/1, BS_Control68/1, BS_Control69/1, BS_Control70/1, BS_Control71/1, BS_Control72/1, BS_Control73/1, BS_Control74/1, BS_Control75/1, BS_Control76/1, BS_Control77/1, BS_Control78/1, BS_Control79/1, BS_Control80/1, BS_Control81/1, BS_Control82/1, BS_Control83/1, BS_Control84/1, BS_Control85/1, BS_Control86/1, BS_Control87/1, BS_Control88/1, BS_Control89/1, BS_Control90/1, BS_Control91/1, BS_Control92/1, BS_Control93/1, BS_Control94/1, BS_Control95/1, BS_Control96/1, BS_Control97/1, BS_Control98/1, BS_Control99/1, BS_Control100/1, BS_Control101/1, BS_Control102/1, BS_Control103/1, BS_Control104/1, BS_Control105/1, BS_Control106/1, BS_Control107/1, BS_Control108/1, BS_Control109/1, BS_Control110/1, BS_Control111/1, BS_Control112/1, BS_Control113/1, BS_Control114/1, BS_Control115/1, BS_Control116/1, BS_Control117/1, BS_Control118/1, BS_Control119/1, BS_Control120/1, BS_Control121/1, BS_Control122/1, BS_Control123/1, BS_Control124/1, BS_Control125/1, BS_Control126/1, BS_Control127/1, BS_Control128/1
  BS_Control1/1 -> EBLR2CB/1(MCBControl)  "<EBLR2CB>"
  Initialise/1 -> EBLR2CB/2(Initialise), EBMVCB/2(Initialise), EDCB/2(Initialise), ELCB1/2(Initialise), ELCB2/2(Initialise), ERCB/2(Initialise), HCB/2(Initialise), HLLCB/2(Initialise), HLRCB/2(Initialise), ILCB1/2(Initialise), ILCB2/2(Initialise), LDICB/2(Initialise), LDLCB/2(Initialise), LDRCB/2(Initialise), MLCB/2(Initialise), MMCB/2(Initialise), NBCB/2(Initialise), NVICB/2(Initialise), OCCB1/2(Initialise), OCCB2/2(Initialise), ODDCB/2(Initialise), PBCB/2(Initialise), PISCB1/2(Initialise), PISCB2/2(Initialise), POCB/2(Initialise), PPU1CB/2(Initialise), PPU2CB/2(Initialise), PPU3CB/2(Initialise), RIO1CB/2(Initialise), RIO2CB/2(Initialise), SIOCB1/2(Initialise), SIOCB2/2(Initialise), SSICB/2(Initialise), TBCCB1/2(Initialise), TBCCB2/2(Initialise), TBNCB/2(Initialise), TDICB/2(Initialise), TLLCB/2(Initialise), TLRCB/2(Initialise), TRIVCB/2(Initialise), TVDUCB/2(Initialise), TWVCB/2(Initialise), VCCBOrUCCB/2(Initialise), VCBCCB/2(Initialise), VIO1CB/2(Initialise), VIO2CB/2(Initialise), WFLCB/2(Initialise), WIFICB/2(Initialise), WWCB/2(Initialise), BECUCB1/2(Initialise), BECUCB2/2(Initialise), BECUCB3/2(Initialise), RSACB/2(Initialise), CMCCB/2(Initialise), CILCB/2(Initialise), CICB/2(Initialise), CELCB/2(Initialise), CECB/2(Initialise), CDUCB/2(Initialise), CCNVIO1CB/2(Initialise), CBTCCB1/2(Initialise), CBFCCB/2(Initialise), CBFCB/2(Initialise), C1CB/2(Initialise), BLCB/2(Initialise), ZVBACB/2(Initialise), EBLR1CB/2(Initialise), DRCB/2(Initialise), DPLCB/2(Initialise), DMICB/2(Initialise), DLCB/2(Initialise), DIOCB2/2(Initialise), DIOCB1/2(Initialise), CSCCB/2(Initialise), CSBCB/2(Initialise), CSACB/2(Initialise), CRSBCB/2(Initialise), SOCB2/2(Initialise), SOCB1/2(Initialise), MSOCB5/2(Initialise), MSOCB4/2(Initialise), MSOCB3/2(Initialise), MSOCB2/2(Initialise), MSOCB1/2(Initialise), HVAC1/2(Initialise), SAC2CCB/2(Initialise), HVAC2/2(Initialise), SAC1CCB/2(Initialise), CMCB/2(Initialise), AC2CB/2(Initialise), AC1CB/2(Initialise), FDSCB/2(Initialise), BCBCB/2(Initialise), ERVRCB1/2(Initialise), ERVRCB2/2(Initialise), ESKCB/2(Initialise), HMCB/2(Initialise), SP1CB/2(Initialise), SP2CB/2(Initialise), SP3CB/2(Initialise), SP4CB/2(Initialise), SP5CB/2(Initialise), SPCB6/2(Initialise), SPCB7/2(Initialise), SPCB8/2(Initialise), RPTCB/2(Initialise), TERCB1/2(Initialise), TERCB2/2(Initialise), SPSW/2(Initialise), SPPB/2(Initialise), APSCB/2(Initialise), APSICB/2(Initialise), BCGCB/2(Initialise), DSCB/2(Initialise), MTBMCCB/2(Initialise), PADCB/2(Initialise), PANCB/2(Initialise), SSCB/2(Initialise), PTCB/2(Initialise), VCBCB/2(Initialise), SP12CB/2(Initialise), MTBM1CB/2(Initialise), MTBM2CB/2(Initialise), SP11CB/2(Initialise), SP6CB/2(Initialise), MTOPCB/2(Initialise), ORDCOS/2(Initialise), ADDCOS/2(Initialise)
  EBLR2CB/1(InputState) -> BC_Inputs/1  "EBLR2CB"
  EBLR2CB/2(MCBTripState) -> BC_MCBTrip/1  "EBLR2CB"
  BS_Control2/1 -> EBMVCB/1(MCBControl)  "<EBMVCB>"
  EBMVCB/1(InputState) -> BC_Inputs/2  "EBMVCB"
  EBMVCB/2(MCBTripState) -> BC_MCBTrip/2  "EBMVCB"
  BS_Control3/1 -> EDCB/1(MCBControl)  "<EDCB>"
  EDCB/1(InputState) -> BC_Inputs/3  "EDCB"
  EDCB/2(MCBTripState) -> BC_MCBTrip/3  "EDCB"
  BS_Control4/1 -> ELCB1/1(MCBControl)  "<ELCB1>"
  ELCB1/1(InputState) -> BC_Inputs/4  "ELCB1"
  ELCB1/2(MCBTripState) -> BC_MCBTrip/4  "ELCB1"
  BS_Control5/1 -> ELCB2/1(MCBControl)  "<ELCB2>"
  ELCB2/1(InputState) -> BC_Inputs/5  "ELCB2"
  ELCB2/2(MCBTripState) -> BC_MCBTrip/5  "ELCB2"
  BS_Control6/1 -> ERCB/1(MCBControl)  "<ERCB>"
  ERCB/1(InputState) -> BC_Inputs/6  "ERCB"
  ERCB/2(MCBTripState) -> BC_MCBTrip/6  "ERCB"
  BS_Control7/1 -> HCB/1(MCBControl)  "<HCB>"
  HCB/1(InputState) -> BC_Inputs/7  "HCB"
  HCB/2(MCBTripState) -> BC_MCBTrip/7  "HCB"
  BS_Control8/1 -> HLLCB/1(MCBControl)  "<HLLCB>"
  HLLCB/1(InputState) -> BC_Inputs/8  "HLLCB"
  HLLCB/2(MCBTripState) -> BC_MCBTrip/8  "HLLCB"
  BS_Control9/1 -> HLRCB/1(MCBControl)  "<HLRCB>"
  HLRCB/1(InputState) -> BC_Inputs/9  "HLRCB"
  HLRCB/2(MCBTripState) -> BC_MCBTrip/9  "HLRCB"
  BS_Control10/1 -> ILCB1/1(MCBControl)  "<ILCB1>"
  ILCB1/1(InputState) -> BC_Inputs/10  "ILCB1"
  ILCB1/2(MCBTripState) -> BC_MCBTrip/10  "ILCB1"
  BS_Control11/1 -> ILCB2/1(MCBControl)  "<ILCB2>"
  ILCB2/1(InputState) -> BC_Inputs/11  "ILCB2"
  ILCB2/2(MCBTripState) -> BC_MCBTrip/11  "ILCB2"
  BS_Control12/1 -> LDICB/1(MCBControl)  "<LDICB>"
  LDICB/1(InputState) -> BC_Inputs/12  "LDICB"
  LDICB/2(MCBTripState) -> BC_MCBTrip/12  "LDICB"
  BS_Control13/1 -> LDLCB/1(MCBControl)  "<LDLCB>"
  LDLCB/1(InputState) -> BC_Inputs/13  "LDLCB"
  LDLCB/2(MCBTripState) -> BC_MCBTrip/13  "LDLCB"
  BS_Control14/1 -> LDRCB/1(MCBControl)  "<LDRCB>"
  LDRCB/1(InputState) -> BC_Inputs/14  "LDRCB"
  LDRCB/2(MCBTripState) -> BC_MCBTrip/14  "LDRCB"
  BS_Control15/1 -> MLCB/1(MCBControl)  "<MLCB>"
  MLCB/1(InputState) -> BC_Inputs/15  "MLCB"
  MLCB/2(MCBTripState) -> BC_MCBTrip/15  "MLCB"
  BS_Control16/1 -> MMCB/1(MCBControl)  "<MMCB>"
  MMCB/1(InputState) -> BC_Inputs/16  "MMCB"
  MMCB/2(MCBTripState) -> BC_MCBTrip/16  "MMCB"
  BS_Control17/1 -> NBCB/1(MCBControl)  "<NBCB>"
  NBCB/1(InputState) -> BC_Inputs/17  "NBCB"
  NBCB/2(MCBTripState) -> BC_MCBTrip/17  "NBCB"
  BS_Control18/1 -> NVICB/1(MCBControl)  "<NVICB>"
  NVICB/1(InputState) -> BC_Inputs/18  "NVICB"
  NVICB/2(MCBTripState) -> BC_MCBTrip/18  "NVICB"
  BS_Control19/1 -> OCCB1/1(MCBControl)  "<OCCB1>"
  OCCB1/1(InputState) -> BC_Inputs/19  "OCCB1"
  OCCB1/2(MCBTripState) -> BC_MCBTrip/19  "OCCB1"
  BS_Control20/1 -> OCCB2/1(MCBControl)  "<OCCB2>"
  OCCB2/1(InputState) -> BC_Inputs/20  "OCCB2"
  OCCB2/2(MCBTripState) -> BC_MCBTrip/20  "OCCB2"
  BS_Control21/1 -> ODDCB/1(MCBControl)  "<ODDCB>"
  ODDCB/1(InputState) -> BC_Inputs/21  "ODDCB"
  ODDCB/2(MCBTripState) -> BC_MCBTrip/21  "ODDCB"
  BS_Control22/1 -> PBCB/1(MCBControl)  "<PBCB>"
  PBCB/1(InputState) -> BC_Inputs/22  "PBCB"
  PBCB/2(MCBTripState) -> BC_MCBTrip/22  "PBCB"
  BS_Control23/1 -> PISCB1/1(MCBControl)  "<PISCB1>"
  PISCB1/1(InputState) -> BC_Inputs/23  "PISCB1"
  PISCB1/2(MCBTripState) -> BC_MCBTrip/23  "PISCB1"
  BS_Control24/1 -> PISCB2/1(MCBControl)  "<PISCB2>"
  PISCB2/1(InputState) -> BC_Inputs/24  "PISCB2"
  PISCB2/2(MCBTripState) -> BC_MCBTrip/24  "PISCB2"
  BS_Control25/1 -> POCB/1(MCBControl)  "<POCB>"
  POCB/1(InputState) -> BC_Inputs/25  "POCB"
  POCB/2(MCBTripState) -> BC_MCBTrip/25  "POCB"
  BS_Control26/1 -> PPU1CB/1(MCBControl)  "<PPU1CB>"
  PPU1CB/1(InputState) -> BC_Inputs/26  "PPU1CB"
  PPU1CB/2(MCBTripState) -> BC_MCBTrip/26  "PPU1CB"
  BS_Control27/1 -> PPU2CB/1(MCBControl)  "<PPU2CB>"
  PPU2CB/1(InputState) -> BC_Inputs/27  "PPU2CB"
  PPU2CB/2(MCBTripState) -> BC_MCBTrip/27  "PPU2CB"
  BS_Control28/1 -> PPU3CB/1(MCBControl)  "<PPU3CB>"
  PPU3CB/1(InputState) -> BC_Inputs/28  "PPU3CB"
  PPU3CB/2(MCBTripState) -> BC_MCBTrip/28  "PPU3CB"
  BS_Control29/1 -> RIO1CB/1(MCBControl)  "<RIO1CB>"
  RIO1CB/1(InputState) -> BC_Inputs/29  "RIO1CB"
  RIO1CB/2(MCBTripState) -> BC_MCBTrip/29  "RIO1CB"
  BS_Control30/1 -> RIO2CB/1(MCBControl)  "<RIO2CB>"
  RIO2CB/1(InputState) -> BC_Inputs/30  "RIO2CB"
  RIO2CB/2(MCBTripState) -> BC_MCBTrip/30  "RIO2CB"
  BS_Control31/1 -> SIOCB1/1(MCBControl)  "<SIOCB1>"
  SIOCB1/1(InputState) -> BC_Inputs/31  "SIOCB1"
  SIOCB1/2(MCBTripState) -> BC_MCBTrip/31  "SIOCB1"
  BS_Control32/1 -> SIOCB2/1(MCBControl)  "<SIOCB2>"
  SIOCB2/1(InputState) -> BC_Inputs/32  "SIOCB2"
  SIOCB2/2(MCBTripState) -> BC_MCBTrip/32  "SIOCB2"
  BS_Control33/1 -> SSICB/1(MCBControl)  "<SSICB>"
  SSICB/1(InputState) -> BC_Inputs/33  "SSICB"
  SSICB/2(MCBTripState) -> BC_MCBTrip/33  "SSICB"
  BS_Control34/1 -> TBCCB1/1(MCBControl)  "<TBCCB1>"
  TBCCB1/1(InputState) -> BC_Inputs/34  "TBCCB1"
  TBCCB1/2(MCBTripState) -> BC_MCBTrip/34  "TBCCB1"
  BS_Control35/1 -> TBCCB2/1(MCBControl)  "<TBCCB2>"
  TBCCB2/1(InputState) -> BC_Inputs/35  "TBCCB2"
  TBCCB2/2(MCBTripState) -> BC_MCBTrip/35  "TBCCB2"
  BS_Control36/1 -> TBNCB/1(MCBControl)  "<TBNCB>"
  TBNCB/1(InputState) -> BC_Inputs/36  "TBNCB"
  TBNCB/2(MCBTripState) -> BC_MCBTrip/36  "TBNCB"
  BS_Control37/1 -> TDICB/1(MCBControl)  "<TDICB>"
  TDICB/1(InputState) -> BC_Inputs/37  "TDICB"
  TDICB/2(MCBTripState) -> BC_MCBTrip/37  "TDICB"
  BS_Control38/1 -> TLLCB/1(MCBControl)  "<TLLCB>"
  TLLCB/1(InputState) -> BC_Inputs/38  "TLLCB"
  TLLCB/2(MCBTripState) -> BC_MCBTrip/38  "TLLCB"
  BS_Control39/1 -> TLRCB/1(MCBControl)  "<TLRCB>"
  TLRCB/1(InputState) -> BC_Inputs/39  "TLRCB"
  TLRCB/2(MCBTripState) -> BC_MCBTrip/39  "TLRCB"
  BS_Control40/1 -> TRIVCB/1(MCBControl)  "<TRIVCB>"
  TRIVCB/1(InputState) -> BC_Inputs/40  "TRIVCB"
  TRIVCB/2(MCBTripState) -> BC_MCBTrip/40  "TRIVCB"
  BS_Control41/1 -> TVDUCB/1(MCBControl)  "<TVDUCB>"
  TVDUCB/1(InputState) -> BC_Inputs/41  "TVDUCB"
  TVDUCB/2(MCBTripState) -> BC_MCBTrip/41  "TVDUCB"
  BS_Control42/1 -> TWVCB/1(MCBControl)  "<TWVCB>"
  TWVCB/1(InputState) -> BC_Inputs/42  "TWVCB"
  TWVCB/2(MCBTripState) -> BC_MCBTrip/42  "TWVCB"
  BS_Control43/1 -> VCCBOrUCCB/1(MCBControl)  "<VCCBOrUCCB>"
  VCCBOrUCCB/1(InputState) -> BC_Inputs/43  "VCCBOrUCCB"
  VCCBOrUCCB/2(MCBTripState) -> BC_MCBTrip/43  "VCCBOrUCCB"
  BS_Control44/1 -> VCBCCB/1(MCBControl)  "<VCBCCB>"
  VCBCCB/1(InputState) -> BC_Inputs/44  "VCBCCB"
  VCBCCB/2(MCBTripState) -> BC_MCBTrip/44  "VCBCCB"
  BS_Control45/1 -> VIO1CB/1(MCBControl)  "<VIO1CB>"
  VIO1CB/1(InputState) -> BC_Inputs/45  "VIO1CB"
  VIO1CB/2(MCBTripState) -> BC_MCBTrip/45  "VIO1CB"
  BS_Control46/1 -> VIO2CB/1(MCBControl)  "<VIO2CB>"
  VIO2CB/1(InputState) -> BC_Inputs/46  "VIO2CB"
  VIO2CB/2(MCBTripState) -> BC_MCBTrip/46  "VIO2CB"
  BS_Control47/1 -> WFLCB/1(MCBControl)  "<WFLCB>"
  WFLCB/1(InputState) -> BC_Inputs/47  "WFLCB"
  WFLCB/2(MCBTripState) -> BC_MCBTrip/47  "WFLCB"
  BS_Control48/1 -> WIFICB/1(MCBControl)  "<WIFICB>"
  WIFICB/1(InputState) -> BC_Inputs/48  "WIFICB"
  WIFICB/2(MCBTripState) -> BC_MCBTrip/48  "WIFICB"
  BS_Control49/1 -> WWCB/1(MCBControl)  "<WWCB>"
  WWCB/1(InputState) -> BC_Inputs/49  "WWCB"
  WWCB/2(MCBTripState) -> BC_MCBTrip/49  "WWCB"
  BS_Control50/1 -> BECUCB1/1(MCBControl)  "<BECUCB1>"
  BECUCB1/1(InputState) -> BC_Inputs/50  "BECUCB1"
  BECUCB1/2(MCBTripState) -> BC_MCBTrip/50  "BECUCB1"
  BS_Control51/1 -> BECUCB2/1(MCBControl)  "<BECUCB2>"
  BECUCB2/1(InputState) -> BC_Inputs/51  "BECUCB2"
  BECUCB2/2(MCBTripState) -> BC_MCBTrip/51  "BECUCB2"
  BS_Control52/1 -> BECUCB3/1(MCBControl)  "<BECUCB3>"
  BECUCB3/1(InputState) -> BC_Inputs/52  "BECUCB3"
  BECUCB3/2(MCBTripState) -> BC_MCBTrip/52  "BECUCB3"
  BS_Control53/1 -> RSACB/1(MCBControl)  "<RSACB>"
  RSACB/1(InputState) -> BC_Inputs/53  "RSACB"
  RSACB/2(MCBTripState) -> BC_MCBTrip/53  "RSACB"
  BS_Control54/1 -> CMCCB/1(MCBControl)  "<CMCCB>"
  CMCCB/1(InputState) -> BC_Inputs/54  "CMCCB"
  CMCCB/2(MCBTripState) -> BC_MCBTrip/54  "CMCCB"
  BS_Control55/1 -> CILCB/1(MCBControl)  "<CILCB>"
  CILCB/1(InputState) -> BC_Inputs/55  "CILCB"
  CILCB/2(MCBTripState) -> BC_MCBTrip/55  "CILCB"
  BS_Control56/1 -> CICB/1(MCBControl)  "<CICB>"
  CICB/1(InputState) -> BC_Inputs/56  "CICB"
  CICB/2(MCBTripState) -> BC_MCBTrip/56  "CICB"
  BS_Control57/1 -> CELCB/1(MCBControl)  "<CELCB>"
  CELCB/1(InputState) -> BC_Inputs/57  "CELCB"
  CELCB/2(MCBTripState) -> BC_MCBTrip/57  "CELCB"
  BS_Control58/1 -> CECB/1(MCBControl)  "<CECB>"
  CECB/1(InputState) -> BC_Inputs/58  "CECB"
  CECB/2(MCBTripState) -> BC_MCBTrip/58  "CECB"
  BS_Control59/1 -> CDUCB/1(MCBControl)  "<CDUCB>"
  CDUCB/1(InputState) -> BC_Inputs/59  "CDUCB"
  CDUCB/2(MCBTripState) -> BC_MCBTrip/59  "CDUCB"
  BS_Control60/1 -> CCNVIO1CB/1(MCBControl)  "<CCNVIO1CB>"
  CCNVIO1CB/1(InputState) -> BC_Inputs/60  "CCNVIO1CB"
  CCNVIO1CB/2(MCBTripState) -> BC_MCBTrip/60  "CCNVIO1CB"
  BS_Control61/1 -> CBTCCB1/1(MCBControl)  "<CBTCCB1>"
  CBTCCB1/1(InputState) -> BC_Inputs/61  "CBTCCB1"
  CBTCCB1/2(MCBTripState) -> BC_MCBTrip/61  "CBTCCB1"
  BS_Control62/1 -> CBFCCB/1(MCBControl)  "<CBFCCB>"
  CBFCCB/1(InputState) -> BC_Inputs/62  "CBFCCB"
  CBFCCB/2(MCBTripState) -> BC_MCBTrip/62  "CBFCCB"
  BS_Control63/1 -> CBFCB/1(MCBControl)  "<CBFCB>"
  CBFCB/1(InputState) -> BC_Inputs/63  "CBFCB"
  CBFCB/2(MCBTripState) -> BC_MCBTrip/63  "CBFCB"
  BS_Control64/1 -> C1CB/1(MCBControl)  "<C1CB>"
  C1CB/1(InputState) -> BC_Inputs/64  "C1CB"
  C1CB/2(MCBTripState) -> BC_MCBTrip/64  "C1CB"
  BS_Control65/1 -> BLCB/1(MCBControl)  "<BLCB>"
  BLCB/1(InputState) -> BC_Inputs/65  "BLCB"
  BLCB/2(MCBTripState) -> BC_MCBTrip/65  "BLCB"
  BS_Control66/1 -> ZVBACB/1(MCBControl)  "<ZVBACB>"
  ZVBACB/1(InputState) -> BC_Inputs/66  "ZVBACB"
  ZVBACB/2(MCBTripState) -> BC_MCBTrip/66  "ZVBACB"
  BS_Control67/1 -> EBLR1CB/1(MCBControl)  "<EBLR1CB>"
  EBLR1CB/1(InputState) -> BC_Inputs/67  "EBLR1CB"
  EBLR1CB/2(MCBTripState) -> BC_MCBTrip/67  "EBLR1CB"
  BS_Control68/1 -> DRCB/1(MCBControl)  "<DRCB>"
  DRCB/1(InputState) -> BC_Inputs/68  "DRCB"
  DRCB/2(MCBTripState) -> BC_MCBTrip/68  "DRCB"
  BS_Control69/1 -> DPLCB/1(MCBControl)  "<DPLCB>"
  DPLCB/1(InputState) -> BC_Inputs/69  "DPLCB"
  DPLCB/2(MCBTripState) -> BC_MCBTrip/69  "DPLCB"
  BS_Control70/1 -> DMICB/1(MCBControl)  "<DMICB>"
  DMICB/1(InputState) -> BC_Inputs/70  "DMICB"
  DMICB/2(MCBTripState) -> BC_MCBTrip/70  "DMICB"
  BS_Control71/1 -> DLCB/1(MCBControl)  "<DLCB>"
  DLCB/1(InputState) -> BC_Inputs/71  "DLCB"
  DLCB/2(MCBTripState) -> BC_MCBTrip/71  "DLCB"
  BS_Control72/1 -> DIOCB2/1(MCBControl)  "<DIOCB2>"
  DIOCB2/1(InputState) -> BC_Inputs/72  "DIOCB2"
  DIOCB2/2(MCBTripState) -> BC_MCBTrip/72  "DIOCB2"
  BS_Control73/1 -> DIOCB1/1(MCBControl)  "<DIOCB1>"
  DIOCB1/1(InputState) -> BC_Inputs/73  "DIOCB1"
  DIOCB1/2(MCBTripState) -> BC_MCBTrip/73  "DIOCB1"
  BS_Control74/1 -> CSCCB/1(MCBControl)  "<CSCCB>"
  CSCCB/1(InputState) -> BC_Inputs/74  "CSCCB"
  CSCCB/2(MCBTripState) -> BC_MCBTrip/74  "CSCCB"
  BS_Control75/1 -> CSBCB/1(MCBControl)  "<CSBCB>"
  CSBCB/1(InputState) -> BC_Inputs/75  "CSBCB"
  CSBCB/2(MCBTripState) -> BC_MCBTrip/75  "CSBCB"
  BS_Control76/1 -> CSACB/1(MCBControl)  "<CSACB>"
  CSACB/1(InputState) -> BC_Inputs/76  "CSACB"
  CSACB/2(MCBTripState) -> BC_MCBTrip/76  "CSACB"
  BS_Control77/1 -> CRSBCB/1(MCBControl)  "<CRSBCB>"
  CRSBCB/1(InputState) -> BC_Inputs/77  "CRSBCB"
  CRSBCB/2(MCBTripState) -> BC_MCBTrip/77  "CRSBCB"
  BS_Control78/1 -> SOCB2/1(MCBControl)  "<SOCB2>"
  SOCB2/1(InputState) -> BC_Inputs/78  "SOCB2"
  SOCB2/2(MCBTripState) -> BC_MCBTrip/78  "SOCB2"
  BS_Control79/1 -> SOCB1/1(MCBControl)  "<SOCB1>"
  SOCB1/1(InputState) -> BC_Inputs/79  "SOCB1"
  SOCB1/2(MCBTripState) -> BC_MCBTrip/79  "SOCB1"
  BS_Control80/1 -> MSOCB5/1(MCBControl)  "<MSOCB5>"
  MSOCB5/1(InputState) -> BC_Inputs/80  "MSOCB5"
  MSOCB5/2(MCBTripState) -> BC_MCBTrip/80  "MSOCB5"
  BS_Control81/1 -> MSOCB4/1(MCBControl)  "<MSOCB4>"
  MSOCB4/1(InputState) -> BC_Inputs/81  "MSOCB4"
  MSOCB4/2(MCBTripState) -> BC_MCBTrip/81  "MSOCB4"
  BS_Control82/1 -> MSOCB3/1(MCBControl)  "<MSOCB3>"
  MSOCB3/1(InputState) -> BC_Inputs/82  "MSOCB3"
  MSOCB3/2(MCBTripState) -> BC_MCBTrip/82  "MSOCB3"
  BS_Control83/1 -> MSOCB2/1(MCBControl)  "<MSOCB2>"
  MSOCB2/1(InputState) -> BC_Inputs/83  "MSOCB2"
  MSOCB2/2(MCBTripState) -> BC_MCBTrip/83  "MSOCB2"
  BS_Control84/1 -> MSOCB1/1(MCBControl)  "<MSOCB1>"
  MSOCB1/1(InputState) -> BC_Inputs/84  "MSOCB1"
  MSOCB1/2(MCBTripState) -> BC_MCBTrip/84  "MSOCB1"
  BS_Control85/1 -> HVAC1/1(MCBControl)  "<HVAC1>"
  HVAC1/1(InputState) -> BC_Inputs/85  "HVAC1"
  HVAC1/2(MCBTripState) -> BC_MCBTrip/85  "HVAC1"
  BS_Control86/1 -> SAC2CCB/1(MCBControl)  "<SAC2CCB>"
  SAC2CCB/1(InputState) -> BC_Inputs/86  "SAC2CCB"
  SAC2CCB/2(MCBTripState) -> BC_MCBTrip/86  "SAC2CCB"
  BS_Control87/1 -> HVAC2/1(MCBControl)  "<HVAC2>"
  HVAC2/1(InputState) -> BC_Inputs/87  "HVAC2"
  HVAC2/2(MCBTripState) -> BC_MCBTrip/87  "HVAC2"
  BS_Control88/1 -> SAC1CCB/1(MCBControl)  "<SAC1CCB>"
  SAC1CCB/1(InputState) -> BC_Inputs/88  "SAC1CCB"
  SAC1CCB/2(MCBTripState) -> BC_MCBTrip/88  "SAC1CCB"
  BS_Control89/1 -> CMCB/1(MCBControl)  "<CMCB>"
  CMCB/1(InputState) -> BC_Inputs/89  "CMCB"
  CMCB/2(MCBTripState) -> BC_MCBTrip/89  "CMCB"
  BS_Control90/1 -> AC2CB/1(MCBControl)  "<AC2CB>"
  AC2CB/1(InputState) -> BC_Inputs/90  "AC2CB"
  AC2CB/2(MCBTripState) -> BC_MCBTrip/90  "AC2CB"
  BS_Control91/1 -> AC1CB/1(MCBControl)  "<AC1CB>"
  AC1CB/1(InputState) -> BC_Inputs/91  "AC1CB"
  AC1CB/2(MCBTripState) -> BC_MCBTrip/91  "AC1CB"
  BS_Control92/1 -> FDSCB/1(MCBControl)  "<FDSCB>"
  FDSCB/1(InputState) -> BC_Inputs/92  "FDSCB"
  FDSCB/2(MCBTripState) -> BC_MCBTrip/92  "FDSCB"
  BS_Control93/1 -> BCBCB/1(MCBControl)  "<BCBCB>"
  BCBCB/1(InputState) -> BC_Inputs/93  "BCBCB"
  BCBCB/2(MCBTripState) -> BC_MCBTrip/93  "BCBCB"
  BS_Control94/1 -> ERVRCB1/1(MCBControl)  "<ERVRCB1>"
  ERVRCB1/1(InputState) -> BC_Inputs/94  "ERVRCB1"
  ERVRCB1/2(MCBTripState) -> BC_MCBTrip/94  "ERVRCB1"
  BS_Control95/1 -> ERVRCB2/1(MCBControl)  "<ERVRCB2>"
  ERVRCB2/1(InputState) -> BC_Inputs/95  "ERVRCB2"
  ERVRCB2/2(MCBTripState) -> BC_MCBTrip/95  "ERVRCB2"
  BS_Control96/1 -> ESKCB/1(MCBControl)  "<ESKCB>"
  ESKCB/1(InputState) -> BC_Inputs/96  "ESKCB"
  ESKCB/2(MCBTripState) -> BC_MCBTrip/96  "ESKCB"
  BS_Control97/1 -> HMCB/1(MCBControl)  "<HMCB>"
  HMCB/1(InputState) -> BC_Inputs/97  "HMCB"
  HMCB/2(MCBTripState) -> BC_MCBTrip/97  "HMCB"
  BS_Control98/1 -> SP1CB/1(MCBControl)  "<SP1CB>"
  SP1CB/1(InputState) -> BC_Inputs/98  "SP1CB"
  SP1CB/2(MCBTripState) -> BC_MCBTrip/98  "SP1CB"
  BS_Control99/1 -> SP2CB/1(MCBControl)  "<SP2CB>"
  SP2CB/1(InputState) -> BC_Inputs/99  "SP2CB"
  SP2CB/2(MCBTripState) -> BC_MCBTrip/99  "SP2CB"
  BS_Control100/1 -> SP3CB/1(MCBControl)  "<SP3CB>"
  SP3CB/1(InputState) -> BC_Inputs/100  "SP3CB"
  SP3CB/2(MCBTripState) -> BC_MCBTrip/100  "SP3CB"
  BS_Control101/1 -> SP4CB/1(MCBControl)  "<SP4CB>"
  SP4CB/1(InputState) -> BC_Inputs/101  "SP4CB"
  SP4CB/2(MCBTripState) -> BC_MCBTrip/101  "SP4CB"
  BS_Control102/1 -> SP5CB/1(MCBControl)  "<SP5CB>"
  SP5CB/1(InputState) -> BC_Inputs/102  "SP5CB"
  SP5CB/2(MCBTripState) -> BC_MCBTrip/102  "SP5CB"
  BS_Control103/1 -> SPCB6/1(MCBControl)  "<SPCB6>"
  SPCB6/1(InputState) -> BC_Inputs/103  "SPCB6"
  SPCB6/2(MCBTripState) -> BC_MCBTrip/103  "SPCB6"
  BS_Control104/1 -> SPCB7/1(MCBControl)  "<SPCB7>"
  SPCB7/1(InputState) -> BC_Inputs/104  "SPCB7"
  SPCB7/2(MCBTripState) -> BC_MCBTrip/104  "SPCB7"
  BS_Control105/1 -> SPCB8/1(MCBControl)  "<SPCB8>"
  SPCB8/1(InputState) -> BC_Inputs/105  "SPCB8"
  SPCB8/2(MCBTripState) -> BC_MCBTrip/105  "SPCB8"
  BS_Control106/1 -> RPTCB/1(MCBControl)  "<RPTCB>"
  RPTCB/1(InputState) -> BC_Inputs/106  "RPTCB"
  RPTCB/2(MCBTripState) -> BC_MCBTrip/106  "RPTCB"
  BS_Control107/1 -> TERCB1/1(MCBControl)  "<TERCB1>"
  TERCB1/1(InputState) -> BC_Inputs/107  "TERCB1"
  TERCB1/2(MCBTripState) -> BC_MCBTrip/107  "TERCB1"
  BS_Control108/1 -> TERCB2/1(MCBControl)  "<TERCB2>"
  TERCB2/1(InputState) -> BC_Inputs/108  "TERCB2"
  TERCB2/2(MCBTripState) -> BC_MCBTrip/108  "TERCB2"
  BS_Control109/1 -> SPSW/1(InputControl)  "<SPSW>"
  SPSW/1(InputState) -> BC_Inputs/109  "SPSW"
  BS_Control110/1 -> SPPB/1(InputControl)  "<SPPB>"
  SPPB/1(InputState) -> BC_Inputs/110  "SPPB"
  BS_Control111/1 -> APSCB/1(MCBControl)  "<APSCB>"
  APSCB/1(InputState) -> BC_Inputs/111  "APSCB"
  APSCB/2(MCBTripState) -> BC_MCBTrip/109  "APSCB"
  BS_Control112/1 -> APSICB/1(MCBControl)  "<APSICB>"
  APSICB/1(InputState) -> BC_Inputs/112  "APSICB"
  APSICB/2(MCBTripState) -> BC_MCBTrip/110  "APSICB"
  BS_Control113/1 -> BCGCB/1(MCBControl)  "<BCGCB>"
  BCGCB/1(InputState) -> BC_Inputs/113  "BCGCB"
  BCGCB/2(MCBTripState) -> BC_MCBTrip/111  "BCGCB"
  BS_Control114/1 -> DSCB/1(MCBControl)  "<DSCB>"
  DSCB/1(InputState) -> BC_Inputs/114  "DSCB"
  DSCB/2(MCBTripState) -> BC_MCBTrip/112  "DSCB"
  BS_Control115/1 -> MTBMCCB/1(MCBControl)  "<MTBMCCB>"
  MTBMCCB/1(InputState) -> BC_Inputs/115  "MTBMCCB"
  MTBMCCB/2(MCBTripState) -> BC_MCBTrip/113  "MTBMCCB"
  BS_Control116/1 -> PADCB/1(MCBControl)  "<PADCB>"
  PADCB/1(InputState) -> BC_Inputs/116  "PADCB"
  PADCB/2(MCBTripState) -> BC_MCBTrip/114  "PADCB"
  BS_Control117/1 -> PANCB/1(MCBControl)  "<PANCB>"
  PANCB/1(InputState) -> BC_Inputs/117  "PANCB"
  PANCB/2(MCBTripState) -> BC_MCBTrip/115  "PANCB"
  BS_Control118/1 -> SSCB/1(MCBControl)  "<SSCB>"
  SSCB/1(InputState) -> BC_Inputs/118  "SSCB"
  SSCB/2(MCBTripState) -> BC_MCBTrip/116  "SSCB"
  BS_Control119/1 -> PTCB/1(MCBControl)  "<PTCB>"
  PTCB/1(InputState) -> BC_Inputs/119  "PTCB"
  PTCB/2(MCBTripState) -> BC_MCBTrip/117  "PTCB"
  BS_Control120/1 -> VCBCB/1(MCBControl)  "<VCBCB>"
  VCBCB/1(InputState) -> BC_Inputs/120  "VCBCB"
  VCBCB/2(MCBTripState) -> BC_MCBTrip/118  "VCBCB"
  BS_Control121/1 -> SP12CB/1(MCBControl)  "<SP12CB>"
  SP12CB/1(InputState) -> BC_Inputs/121  "SP12CB"
  SP12CB/2(MCBTripState) -> BC_MCBTrip/119  "SP12CB"
  BS_Control122/1 -> MTBM1CB/1(MCBControl)  "<MTBM1CB>"
  MTBM1CB/1(InputState) -> BC_Inputs/122  "MTBM1CB"
  MTBM1CB/2(MCBTripState) -> BC_MCBTrip/120  "MTBM1CB"
  BS_Control123/1 -> MTBM2CB/1(MCBControl)  "<MTBM2CB>"
  MTBM2CB/1(InputState) -> BC_Inputs/123  "MTBM2CB"
  MTBM2CB/2(MCBTripState) -> BC_MCBTrip/121  "MTBM2CB"
  BS_Control124/1 -> SP11CB/1(MCBControl)  "<SP11CB>"
  SP11CB/1(InputState) -> BC_Inputs/124  "SP11CB"
  SP11CB/2(MCBTripState) -> BC_MCBTrip/122  "SP11CB"
  BS_Control125/1 -> SP6CB/1(MCBControl)  "<SP6CB>"
  SP6CB/1(InputState) -> BC_Inputs/125  "SP6CB"
  SP6CB/2(MCBTripState) -> BC_MCBTrip/123  "SP6CB"
  BS_Control126/1 -> MTOPCB/1(MCBControl)  "<MTOPCB>"
  MTOPCB/1(InputState) -> BC_Inputs/126  "MTOPCB"
  MTOPCB/2(MCBTripState) -> BC_MCBTrip/124  "MTOPCB"
  BS_Control127/1 -> ORDCOS/1(InputControl)  "<ORDCOS>"
  ORDCOS/1(InputState) -> BC_Inputs/127  "ORDCOS"
  BS_Control128/1 -> ADDCOS/1(InputControl)  "<ADDCOS>"
  ADDCOS/1(InputState) -> BC_Inputs/128  "ADDCOS"
